simulink model "Michaels_CVModel_fast8"  (R2020a)
settings: Solver=ode23  StartTime=0.0  StopTime=30  RelTol=1e-2  EnableMultiTasking=on
model workspace (MAT data in the model file):
  Eao = 1.88
  Eesla = 0.58
  Eeslvf = 5.2
  Eesra = 0.63
  Eesrvf = 1.75
  Emaxspt = 48.75
  Epa = 0.15
  Epu = 0.04
  Esa = 0.37
  Esv = 0.013
  Evc = 0.03
  GpLV = 0
  GpRR = 11
  GpRV = 0
  GpRsa = 0
  GpV0 = 0
  GsLV = 0.007
  GsRR = 11
  GsRV = 0.022
  GsRsa = -0.05
  GsV0 = 31
  Ka = 4.4
  Lao = 0.0022
  Lav = 0.000354
  Lmt = 7.697e-05
  Lpa = 7.697e-05
  Lpv = 0.0001043
  Ltc = 8.009e-05
  P0la = 0.5
  P0lvf = 0.98
  P0pcd = 0.5
  P0ra = 0.5
  P0rvf = 0.91
  P0spt = 0.46
  PV : AO (value not decoded)
  PVao = [327.9; 100.9]
  Rao = 0.28
  Rav = 0.02
  Rla2pu = 0.5
  Rmt = 0.01
  Rpa = 0.12
  Rpa_Vals = 0.12
  Rpu = 0.006
  Rpv = 0.02
  Rra = 0.012
  Rsa = 0.74
  Rsv = 0.12
  Rtc = 0.01
  Tc = 1
  Tsys0 = 0.6
  V0la = 30
  V0lvf = 45
  V0pcd = 200
  V0ra = 25
  V0rvf = 50
  V0spt = 10
  Vdla = 15
  Vdlvf = 16
  Vdra = 15
  Vdrvf = 40
  Vdspt = 10
  Vlv0 = 100
  Vperi = 51
  Vrv0 = 105
  Vuao = 260.8
  Vupa = 91
  Vupu = 132
  Vusa = 287.4
  Vusv = 1976.1
  Vuvc = 136.17
  amin = -2
  artBrLVcontConti = []
  artBrLVcontDigi = [0 0 0 0 0 0 0 0 0 0 0 0 ... (240 elements, 1x240)]
  artBrRRConti = []
  artBrRRDigi = [0 0 0 0 0 0 0 0 0 0 1.57142857143 3.14285714286 ... (240 elements, 1x240)]
  artBrRVcontConti = []
  artBrRVcontDigi = [0 0 0 0 0 0 0 0 0 0 0 0 ... (240 elements, 1x240)]
  artBrRsaConti = []
  artBrRsaDigi = [0 0 0 0 0 0 0 0 0 0 0 0 ... (480 elements, 1x480)]
  artBrV0Conti = []
  artBrV0Digi = [0 0 0 0 0 0 0 0 0 0 0 0 ... (640 elements, 1x640)]
  atriumA = 1
  baroSampFreq = 16
  cP0la = 0.5
  cP0lvf = 0.98
  cP0ra = 0.5
  cP0rvf = 0.91
  cT = 1
  cVtotal = 5400
  clambdala = 0.13
  clambdalvf = 0.028
  clambdara = 0.13
  clambdarvf = 0.028
  deac = 0.0004
  ksys = 0.075
  lambdala = 0.065
  lambdalvf = 0.042
  lambdapcd = 0.005
  lambdara = 0.065
  lambdarvf = 0.028
  lambdaspt = 0.4
  pThor = 0
  params : object (value not decoded)
  sampleTime = 0.005
  svcPressureChange_MCS = 0
  svrMult = 1
  tStepOn = 1000000000
  t_baroOn = 1000000
  t_testBed_start = 1000000
  venk1 = 0.5
  venk2 = 0.5
symbols that are objects in the model workspace (value not decoded): PV
undefined symbols (not defined in the file): dfilt
libraries: simulink x85, fl_lib x39, nesl_utility x24, cstblocks x9, dspstat3 x9, dspobslib x5, SimscapeFluids_lib x5, sh_lib x1
(part 4 of 5)

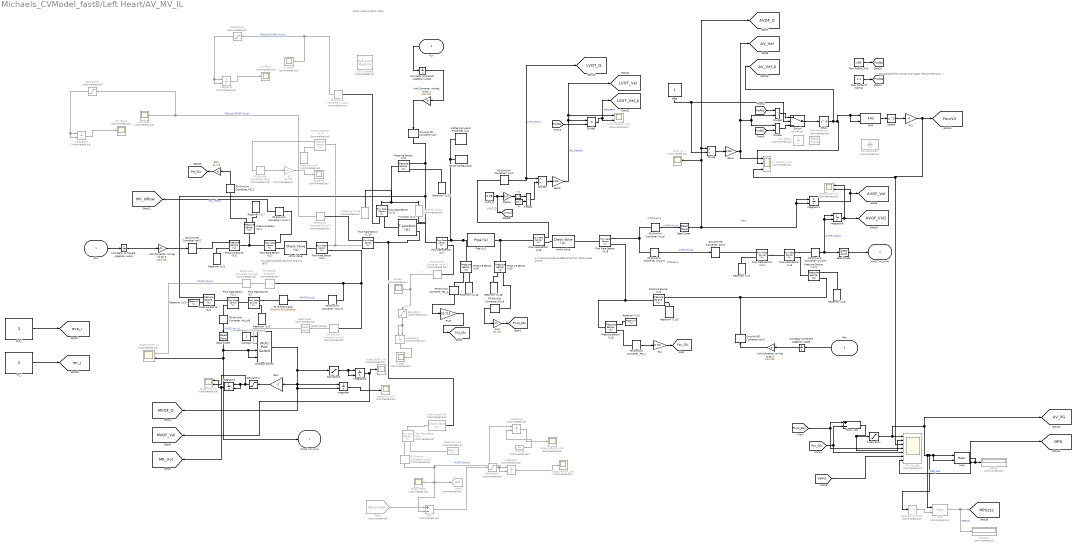
== system Michaels_CVModel_fast8/Left Heart/AV_MV_IL ==
  note: MV opening pressures from Tsakiris 1978
  note: AV cracking pressure differential from 2019 Lansac article
  note: Extrapolated from Donati 2017 paper "Beyond Bernoulli..."
  note: Filtered Q
  note: Unfiltered Q
  note: 1 = Unfiltered Q
      | 2= Filtered Q
  note: Area
  note: Aortic Valve & Mitral Valve
  PLA : Inport
  PLV : Inport  Port=2
  PAo : Inport  Port=3
  4V2 : Gain  Gain=4
  51.1 : Gain  Gain=51.715
  51.7 : Gain  Commented=on  Gain=51.715
  51.8 : Gain  Gain=51.715
  AV Velocity (m/s) : Scope  Commented=on  NumInputPorts=3
  AVOF_Q : Scope  Commented=on
  Add : Sum  Commented=on  Inputs=+-
  Aortic Valve : SimscapeFluids_lib/Isothermal Liquid/Valves & Orifices/Directional Control Valves/Check Valve (IL)  pressure_control_spec=fluids.isothermal_liquid.valves_orifices.enum.pressure_control_spec.dp  p_crack_differential=0.01 psi  p_crack_gauge=0.001 psi  press_max_differential=0.25 psi  press_max_gauge=0.002 psi  area_max=4 cm^2  area_leak=1e-13 cm^2  area=inf cm^2  Cd=0.85  Re_c=8000  pressure_recovery=simscape.enum.onoff.off  opening_dynamics=simscape.enum.onoff.on  tau=10 ms  mdot_A_specify=off  mdot_A_priority=None  mdot_A=0 kg/s  mdot_A_nominal_specify=off  mdot_A_nominal_unit=kg/s  mdot_A_nominal_value=1  mdot_B_specify=off  mdot_B_priority=None  mdot_B=0 kg/s  mdot_B_nominal_specify=off  mdot_B_nominal_unit=kg/s  mdot_B_nominal_value=1
      settings: SourceProductBaseCode=SH  InternalSimscapePortConfiguration="{\"Bottom\":[],\"Left\":[{\"id\":\"A\",\"label\":\"A\",\"type\":\"foundation.isothermal_liquid.isothermal_liquid\"}],\"Right\":[{\"id\":\"B\",\"label\":\"B\",\"type\":\"foundation.isothermal_liquid.isothermal_liquid\"}],\"Top\":[]}"
  Check Valve (MR) : SimscapeFluids_lib/Isothermal Liquid/Valves & Orifices/Directional Control Valves/Check Valve (IL)  Commented=on  pressure_control_spec=fluids.isothermal_liquid.valves_orifices.enum.pressure_control_spec.dp  p_crack_differential=0.001 psi  p_crack_gauge=0.1 MPa  press_max_differential=0.00101 psi  press_max_gauge=0.2 MPa  area_max=0.2 cm^2  area_leak=1e-13 cm^2  area=inf cm^2  Cd=0.9  Re_c=5000  pressure_recovery=simscape.enum.onoff.off  opening_dynamics=simscape.enum.onoff.off  tau=0.1 s  mdot_A_specify=off  mdot_A_priority=None  mdot_A=0 kg/s  mdot_A_nominal_specify=off  mdot_A_nominal_unit=kg/s  mdot_A_nominal_value=1  mdot_B_specify=off  mdot_B_priority=None  mdot_B=0 kg/s  mdot_B_nominal_specify=off  mdot_B_nominal_unit=kg/s  mdot_B_nominal_value=1
      settings: SourceProductBaseCode=SH  InternalSimscapePortConfiguration="{\"Bottom\":[],\"Left\":[{\"id\":\"A\",\"label\":\"A\",\"type\":\"foundation.isothermal_liquid.isothermal_liquid\"}],\"Right\":[{\"id\":\"B\",\"label\":\"B\",\"type\":\"foundation.isothermal_liquid.isothermal_liquid\"}],\"Top\":[]}"
  Compare To Zero1 : simulink/Logic and Bit Operations/Compare To Zero  Commented=on  relop=>  OutDataTypeStr=boolean
  Constant : Constant  Value=2
  Dead Zone2 : DeadZone  Commented=on  LowerValue=-0.01  UpperValue=0.01  SaturateOnIntegerOverflow=on
  Dead Zone3 : DeadZone  LowerValue=-0.001  UpperValue=0.001  ZeroCross=off  SaturateOnIntegerOverflow=on
  Dead Zone4 : DeadZone  LowerValue=-0.001  UpperValue=0.001  ZeroCross=off  SaturateOnIntegerOverflow=on
  Dead Zone5 : DeadZone  LowerValue=-0.001  UpperValue=0.001  ZeroCross=off  SaturateOnIntegerOverflow=on
  Delay : Delay  DelayLength=0  SampleTime=0.001
  Discrete Filter1 : DiscreteFilter  Commented=on  Denominator=[1]  SampleTime=0.001
  Display : Display  Commented=on
  Display1 : Display  Commented=on
  Divide : Product  Inputs=*/
  Divide1 : Product  Inputs=**
  Divide2 : Product  Inputs=*/
  Divide3 : Product  Inputs=**
  Divide4 : Product  Inputs=**
  Flow Profile Cf AS : Constant  Value=1.305  SampleTime=0.001
  Flow Profile Cf Normal : Constant  Value=1.1  SampleTime=0.001
  Flow Rate Sensor (IL){1..3,5,7..11} (9 alike) : fl_lib/Isothermal Liquid/Sensors/Flow Rate Sensor (IL)  sensor_type=foundation.enum.mass_volumetric_sensor.volumetric
      settings: SourceProductBaseCode=SS  InternalSimscapePortConfiguration="{\"Bottom\":[],\"Left\":[{\"id\":\"A\",\"label\":\"A\",\"type\":\"foundation.isothermal_liquid.isothermal_liquid\"}],\"Right\":[{\"id\":\"B\",\"label\":\"B\",\"type\":\"foundation.isothermal_liquid.isothermal_liquid\"},{\"id\":\"V\",\"label\":\"V\",\"type\":\"output\"}],\"Top\":[]}"
  Flow Rate Sensor (IL)6 : fl_lib/Isothermal Liquid/Sensors/Flow Rate Sensor (IL)  Commented=on  sensor_type=foundation.enum.mass_volumetric_sensor.volumetric
      settings: SourceProductBaseCode=SS  InternalSimscapePortConfiguration="{\"Bottom\":[],\"Left\":[{\"id\":\"A\",\"label\":\"A\",\"type\":\"foundation.isothermal_liquid.isothermal_liquid\"}],\"Right\":[{\"id\":\"B\",\"label\":\"B\",\"type\":\"foundation.isothermal_liquid.isothermal_liquid\"},{\"id\":\"V\",\"label\":\"V\",\"type\":\"output\"}],\"Top\":[]}"
  Flow Rate Source (IL) : fl_lib/Isothermal Liquid/Sources/Flow Rate Source (IL)  source_type=foundation.enum.constant_controlled.controlled  flow_type=foundation.enum.mass_volumetric_flow.volumetric  mass_flow=0 kg/s  volumetric_flow=0 m^3/s
      settings: SourceProductBaseCode=SS  InternalSimscapePortConfiguration="{\"Bottom\":[],\"Left\":[{\"id\":\"A\",\"label\":\"A\",\"type\":\"foundation.isothermal_liquid.isothermal_liquid\"},{\"id\":\"V\",\"label\":\"V\",\"type\":\"input\"}],\"Right\":[{\"id\":\"B\",\"label\":\"B\",\"type\":\"foundation.isothermal_liquid.isothermal_liquid\"}],\"Top\":[]}"
  Flow Rate Source (IL)1 : fl_lib/Isothermal Liquid/Sources/Flow Rate Source (IL)  source_type=foundation.enum.constant_controlled.controlled  flow_type=foundation.enum.mass_volumetric_flow.volumetric  mass_flow=0 kg/s  volumetric_flow=0 m^3/s
      settings: SourceProductBaseCode=SS  InternalSimscapePortConfiguration="{\"Bottom\":[],\"Left\":[{\"id\":\"A\",\"label\":\"A\",\"type\":\"foundation.isothermal_liquid.isothermal_liquid\"},{\"id\":\"V\",\"label\":\"V\",\"type\":\"input\"}],\"Right\":[{\"id\":\"B\",\"label\":\"B\",\"type\":\"foundation.isothermal_liquid.isothermal_liquid\"}],\"Top\":[]}"
  From16 : From  Commented=on  GotoTag=ev  TagVisibility=global
      settings: CloseFcn=tagdialog Close
  From2 : From  Commented=on  GotoTag=MV_Inflow  TagVisibility=global
  Gain : Gain  Gain=-1
  Gain1 : Gain  Gain=1/100
  Gain3 : Gain  Gain=1/100
  Goto3 : Goto  Commented=on  GotoTag=QMR  TagVisibility=global
  Integrator{,1..3,9} (5 alike) : Integrator  ExternalReset=either
  Integrator4 : Integrator  Commented=on  ExternalReset=either
  Integrator5 : Integrator  Commented=on  ExternalReset=either
  Integrator6 : Integrator  Commented=on  ExternalReset=rising
  Integrator7 : Integrator  Commented=on  ExternalReset=rising
  Integrator8 : Integrator  Commented=on  ExternalReset=rising
  Isothermal Liquid Properties (IL)1 : fl_lib/Isothermal Liquid/Utilities/Isothermal Liquid Properties (IL)  rho_L_atm=1107.1 kg/m^3  bulk_modulus_model=foundation.enum.bulk_modulus_model.const  beta_gain=6  beta_L_atm=2.1791e9 Pa  nu_atm=3.5 cSt  air_fraction=0  polytropic_index=1.0  rho_g_atm=1.225 kg/m^3  air_dissolution_model=simscape.enum.onoff.off  p_crit=3 MPa  p_atm=14.6959 psi  p_min=1e-13 psi
      settings: SourceProductBaseCode=SS
  LV Inflow2 : Scope  Commented=on
  LV Inflow3 : Scope  Commented=on
  LVOT Velocity (m/s) : Scope  Commented=on  NumInputPorts=2
  LVOT1 -flexible : sh_lib/Pipelines/Hydraulic Pipeline  Commented=on  cs_type=1  d_in=2.0 cm  area=1e-4 m^2  D_h=1.12e-2 m  s_factor=64  length=1.8 cm  length_ad=0.4 cm  roughness=0.1 cm  Re_lam=2000  Re_turb=5000  wall_type=2  pr_r_coef=2e-12 m/Pa  time_const=0.01 s  k_sh=1.4  initial_pressure=0.01 psi
      settings: SourceProductBaseCode=SH  InternalSimscapePortConfiguration="{\"Bottom\":[],\"Left\":[{\"id\":\"A\",\"label\":\"A\",\"type\":\"foundation.hydraulic.hydraulic\"}],\"Right\":[{\"id\":\"B\",\"label\":\"B\",\"type\":\"foundation.hydraulic.hydraulic\"}],\"Top\":[]}"
  LVOT_D : Constant  Value=2.25
  MPG : dspstat3/Mean  run=on  reset_popup=Either edge  directionMode=Each column  dimension=1  roiEnable=off  roiType=Rectangles  roiPortion=Entire ROI  roiOutput=Individual statistics for each ROI  roiFlag=off  roundingMode=Floor  overflowMode=off  outputDataTypeStr=Inherit: Same as accumulator  outputMin=[]  outputMax=[]  outputLastDataTypeStr=Inherit: Same as accumulator
  MPG1 : dspstat3/Mean  Commented=on  run=on  reset_popup=Either edge  directionMode=Each column  dimension=1  roiEnable=off  roiType=Rectangles  roiPortion=Entire ROI  roiOutput=Individual statistics for each ROI  roiFlag=off  roundingMode=Floor  overflowMode=off  outputDataTypeStr=Inherit: Same as accumulator  outputMin=[]  outputMax=[]  outputLastDataTypeStr=Inherit: Same as accumulator
  MR Inflow : Scope  Commented=on
  MR Inflow1 : Scope  Commented=on
  Mitral Valve : SimscapeFluids_lib/Isothermal Liquid/Valves & Orifices/Directional Control Valves/Check Valve (IL)  pressure_control_spec=fluids.isothermal_liquid.valves_orifices.enum.pressure_control_spec.dp  p_crack_differential=0.0001 psi  p_crack_gauge=0.001 psi  press_max_differential=0.15 psi  press_max_gauge=0.002 psi  area_max=5 cm^2  area_leak=1e-13 cm^2  area=3.1416*1.27^2 cm^2  Cd=0.85  Re_c=5000  pressure_recovery=simscape.enum.onoff.off  opening_dynamics=simscape.enum.onoff.on  tau=20 ms  mdot_A_specify=off  mdot_A_priority=None  mdot_A=0 kg/s  mdot_A_nominal_specify=off  mdot_A_nominal_unit=kg/s  mdot_A_nominal_value=1  mdot_B_specify=off  mdot_B_priority=None  mdot_B=0 kg/s  mdot_B_nominal_specify=off  mdot_B_nominal_unit=kg/s  mdot_B_nominal_value=1
      settings: SourceProductBaseCode=SH  InternalSimscapePortConfiguration="{\"Bottom\":[],\"Left\":[{\"id\":\"A\",\"label\":\"A\",\"type\":\"foundation.isothermal_liquid.isothermal_liquid\"}],\"Right\":[{\"id\":\"B\",\"label\":\"B\",\"type\":\"foundation.isothermal_liquid.isothermal_liquid\"}],\"Top\":[]}"
  Multiport Switch : MultiPortSwitch
  P saturation : Saturate  UpperLimit=inf  LowerLimit=0
  PS Transfer Function1 : fl_lib/Physical Signals/Linear Operators/PS Transfer Function  Commented=on  transfer_function_type=foundation.enum.transfer_function_type.lag  T=5 ms  T1=2 s  T2=1 s  y0=100 cm^3/s
      settings: SourceProductBaseCode=SS  InternalSimscapePortConfiguration="{\"Bottom\":[],\"Left\":[{\"id\":\"U\",\"label\":\"\",\"type\":\"input\"}],\"Right\":[{\"id\":\"Y\",\"label\":\"\",\"type\":\"output\"}],\"Top\":[]}"
  PS-Simulink Converter (mL/s){,5,7..9} (5 alike) : nesl_utility/PS-Simulink Converter  PhysicalDomain=network_engine_domain  SubClassName=ps_output  LeftPortType=input  RightPortType=output  PseudoPeriodic=off  Frequencies=[]  Unit=cm^3/s  AffineConversion=off
  "PS-Simulink Converter (mL/s) " : nesl_utility/PS-Simulink Converter  PhysicalDomain=network_engine_domain  SubClassName=ps_output  LeftPortType=input  RightPortType=output  PseudoPeriodic=off  Frequencies=[]  Unit=cm^3/s  AffineConversion=off
  PS-Simulink Converter (mL/s) 1 : nesl_utility/PS-Simulink Converter  Commented=on  PhysicalDomain=network_engine_domain  SubClassName=ps_output  LeftPortType=input  RightPortType=output  PseudoPeriodic=off  Frequencies=[]  Unit=cm^3/s  AffineConversion=off
  PS-Simulink Converter (mL/s) 2 : nesl_utility/PS-Simulink Converter  PhysicalDomain=network_engine_domain  SubClassName=ps_output  LeftPortType=input  RightPortType=output  PseudoPeriodic=off  Frequencies=[]  Unit=cm^3/s  AffineConversion=off
  PS-Simulink Converter (mL/s){1..4,6} (5 alike) : nesl_utility/PS-Simulink Converter  Commented=on  PhysicalDomain=network_engine_domain  SubClassName=ps_output  LeftPortType=input  RightPortType=output  PseudoPeriodic=off  Frequencies=[]  Unit=cm^3/s  AffineConversion=off
  PS-Simulink Converter_PSI_{1..2,4,9} (4 alike) : nesl_utility/PS-Simulink Converter  PhysicalDomain=network_engine_domain  SubClassName=ps_output  LeftPortType=input  RightPortType=output  PseudoPeriodic=off  Frequencies=[]  Unit=psi  AffineConversion=off
  PS-Simulink Converter_PSI_8 : nesl_utility/PS-Simulink Converter  Commented=on  PhysicalDomain=network_engine_domain  SubClassName=ps_output  LeftPortType=input  RightPortType=output  PseudoPeriodic=off  Frequencies=[]  Unit=psi  AffineConversion=off
  Pav : Gain  Gain=51.715
  Pi : Constant  Value=pi()  SampleTime=0.001
  Pipe (IL)1 : SimscapeFluids_lib/Isothermal Liquid/Pipes & Fittings/Pipe (IL)  dynamic_compressibility=simscape.enum.onoff.off  inertia=simscape.enum.onoff.off  num_segments=1  pipe_length=1.8 cm  cross_section_geometry=fluids.isothermal_liquid.pipes_fittings.enum.cross_section_geometry.circular  pipe_diameter=2.25 cm  pipe_inner_diameter=0.05 m  pipe_outer_diameter=0.1 m  pipe_width=0.1 m  pipe_height=0.1 m  pipe_major_axis=0.1 m  pipe_minor_axis=0.05 m  pipe_side=0.1 m  pipe_angle=30 deg  pipe_area=0.01 m^2  Dh=0.1128 m  elevation_spec=foundation.enum.constant_variable.constant  elevation_gain=0 cm  gravity_spec=foundation.enum.constant_variable.constant  g=9.81 m/s^2  pressure_loss_spec=fluids.isothermal_liquid.pipes_fittings.enum.pressure_loss_spec.haaland  mdot_nominal=[.1, 1] kg/s  p_diff_nominal=[.001, .01] MPa  mdot_threshold=1e-6 kg/s  local_pressure_loss_spec=fluids.isothermal_liquid.pipes_fittings.enum.local_loss_spec.aggregate_length  length_add=0.004 cm  loss_coefficient=0.1  roughness_spec=fluids.isothermal_liquid.pipes_fittings.enum.roughness_spec.commercial_pipe  roughness=15e-6 m  Re_friction_TLU=[400, 1000, 1500, 3000, 4000, 6000, 10000, 20000, 40000, 60000, 100000, 100000000]  friction_factor_TLU=[.264, .112, .071, .0417, .0387, .0268, .025, .0232, .0226, .022, .0214, .0214]  Re_lam=5000  Re_tur=8000  shape_factor=64  pipe_wall_spec=fluids.isothermal_liquid.pipes_fittings.enum.wall_spec.flexible  vol_expansion_spec=fluids.isothermal_liquid.pipes_fittings.enum.vol_expansion_spec.area  area_pressure_gain=0.005 m^2/MPa  diameter_pressure_gain=1e-6 m/MPa  wall_time_constant=0.12 s  p0=0.1 psi  mdot0=0 kg/s
      settings: SourceProductBaseCode=SH  InternalSimscapePortConfiguration="{\"Bottom\":[],\"Left\":[{\"id\":\"A\",\"label\":\"A\",\"type\":\"foundation.isothermal_liquid.isothermal_liquid\"}],\"Right\":[{\"id\":\"B\",\"label\":\"B\",\"type\":\"foundation.isothermal_liquid.isothermal_liquid\"}],\"Top\":[]}"
  Plv_Pav_Sat : Scope  Commented=on  NumInputPorts=7
  Plvot : Gain  Gain=51.715
  Plvot - Pav : Sum  Inputs=+-
  Pressure Sensor (IL){1,6,8..9} (4 alike) : fl_lib/Isothermal Liquid/Sensors/Pressure Sensor (IL)  pressure_measure=foundation.enum.pressure_measure.difference
      settings: SourceProductBaseCode=SS  InternalSimscapePortConfiguration="{\"Bottom\":[],\"Left\":[{\"id\":\"A\",\"label\":\"A\",\"type\":\"foundation.isothermal_liquid.isothermal_liquid\"}],\"Right\":[{\"id\":\"B\",\"label\":\"B\",\"type\":\"foundation.isothermal_liquid.isothermal_liquid\"},{\"id\":\"P\",\"label\":\"P\",\"type\":\"output\"}],\"Top\":[]}"
  Pressure Sensor (IL)5 : fl_lib/Isothermal Liquid/Sensors/Pressure Sensor (IL)  Commented=on  pressure_measure=foundation.enum.pressure_measure.difference
      settings: SourceProductBaseCode=SS  InternalSimscapePortConfiguration="{\"Bottom\":[],\"Left\":[{\"id\":\"A\",\"label\":\"A\",\"type\":\"foundation.isothermal_liquid.isothermal_liquid\"}],\"Right\":[{\"id\":\"B\",\"label\":\"B\",\"type\":\"foundation.isothermal_liquid.isothermal_liquid\"},{\"id\":\"P\",\"label\":\"P\",\"type\":\"output\"}],\"Top\":[]}"
  Pressure Source (IL){1..5} (5 alike) : fl_lib/Isothermal Liquid/Sources/Pressure Source (IL)  source_type=foundation.enum.constant_controlled.controlled  pressure_differential=0 MPa
      settings: SourceProductBaseCode=SS  InternalSimscapePortConfiguration="{\"Bottom\":[],\"Left\":[{\"id\":\"A\",\"label\":\"A\",\"type\":\"foundation.isothermal_liquid.isothermal_liquid\"},{\"id\":\"P\",\"label\":\"P\",\"type\":\"input\"}],\"Right\":[{\"id\":\"B\",\"label\":\"B\",\"type\":\"foundation.isothermal_liquid.isothermal_liquid\"}],\"Top\":[]}"
  Product : Product
  RMS : dspstat3/RMS  run=on  directionMode=Each column  dimension=1  reset_popup=Either edge
  Radius : Gain  Gain=0.5
  Rate Transition2 : RateTransition  Commented=on
  Reservoir (IL){1..7,13,15,18..19} (11 alike) : fl_lib/Isothermal Liquid/Elements/Reservoir (IL)  reservoir_type=foundation.enum.constant_controlled.constant  pressure_spec=foundation.enum.pressure_spec.atmospheric  reservoir_pressure=0.101325 MPa
      settings: SourceProductName=Foundation Library
  Reservoir (IL)11 : fl_lib/Isothermal Liquid/Elements/Reservoir (IL)  Commented=on  reservoir_type=foundation.enum.constant_controlled.controlled  pressure_spec=foundation.enum.pressure_spec.atmospheric  reservoir_pressure=0.101325 MPa
      settings: SourceProductName=Foundation Library  InternalSimscapePortConfiguration="{\"Bottom\":[],\"Left\":[{\"id\":\"A\",\"label\":\"A\",\"type\":\"foundation.isothermal_liquid.isothermal_liquid\"}],\"Right\":[{\"id\":\"P\",\"label\":\"P\",\"type\":\"input\"}],\"Top\":[]}"
  Reservoir (IL)16 : fl_lib/Isothermal Liquid/Elements/Reservoir (IL)  Commented=on  reservoir_type=foundation.enum.constant_controlled.constant  pressure_spec=foundation.enum.pressure_spec.atmospheric  reservoir_pressure=0.101325 MPa
      settings: SourceProductName=Foundation Library
  Reservoir (IL)8 : fl_lib/Isothermal Liquid/Elements/Reservoir (IL)  Commented=on  reservoir_type=foundation.enum.constant_controlled.constant  pressure_spec=foundation.enum.pressure_spec.atmospheric  reservoir_pressure=0.101325 MPa
      settings: SourceProductName=Foundation Library
  Reservoir (IL)9 : fl_lib/Isothermal Liquid/Elements/Reservoir (IL)  Commented=on  reservoir_type=foundation.enum.constant_controlled.constant  pressure_spec=foundation.enum.pressure_spec.atmospheric  reservoir_pressure=0.101325 MPa
      settings: SourceProductName=Foundation Library
  Saturation1 : Saturate  UpperLimit=inf  LowerLimit=0
  Saturation2 : Saturate  UpperLimit=inf  LowerLimit=0
  Saturation{5..7,9} (4 alike) : Saturate  Commented=on  UpperLimit=inf  LowerLimit=0
  Scope1 : Scope  Commented=on
  Scope3 : Scope  Commented=on
  Scope_AVOF_Vol : Scope  Commented=on  NumInputPorts=2
  Scope_MROF : Scope  Commented=on
  Scope_MRVOF_Vol1 : Scope  Commented=on
  Scope_MRVOF_Vol2 : Scope  Commented=on
  Scope_MR_Vol : Scope  Commented=on  NumInputPorts=2
  Scope_MVOF_Q : Scope  Commented=on  NumInputPorts=2
  Scope_MVOF_Vol : Scope  Commented=on
  Scope_MV_Vol2 : Scope  Commented=on
  Scope_P1 : Scope  Commented=on
  Simulink-PS Converter (psi) : nesl_utility/Simulink-PS Converter  PhysicalDomain=network_engine_domain  SubClassName=ps_input  LeftPortType=input  RightPortType=output  PseudoPeriodic=off  Frequencies=[]  NoiseDistribution=none  NoiseParameters=[]  Unit=psi  AffineConversion=off  FilteringAndDerivatives=filter  SimscapeFilterOrder=1  InputFilterTimeConstant=.001  UdotUserProvided=0
  Simulink-PS Converter (psi)1 : nesl_utility/Simulink-PS Converter  PhysicalDomain=network_engine_domain  SubClassName=ps_input  LeftPortType=input  RightPortType=output  PseudoPeriodic=off  Frequencies=[]  NoiseDistribution=none  NoiseParameters=[]  Unit=psi  AffineConversion=off  FilteringAndDerivatives=filter  SimscapeFilterOrder=1  InputFilterTimeConstant=.001  UdotUserProvided=0
  Simulink-PS Converter (psi)2 : nesl_utility/Simulink-PS Converter  PhysicalDomain=network_engine_domain  SubClassName=ps_input  LeftPortType=input  RightPortType=output  PseudoPeriodic=off  Frequencies=[]  NoiseDistribution=none  NoiseParameters=[]  Unit=psi  AffineConversion=off  FilteringAndDerivatives=filter  SimscapeFilterOrder=1  InputFilterTimeConstant=.001  UdotUserProvided=0
  Simulink-PS Converter (psi)5 : nesl_utility/Simulink-PS Converter  PhysicalDomain=network_engine_domain  SubClassName=ps_input  LeftPortType=input  RightPortType=output  PseudoPeriodic=off  Frequencies=[]  NoiseDistribution=none  NoiseParameters=[]  Unit=cm^3/s  AffineConversion=off  FilteringAndDerivatives=filter  SimscapeFilterOrder=1  InputFilterTimeConstant=.002  UdotUserProvided=0
  "Solver Configuration " : nesl_utility/Solver Configuration  PhysicalDomain=network_engine_domain  SubClassName=solver  LeftPortType=input  RightPortType=generic  Tones=[]  Harmonics=[]  SimulateNoise=off  Profile=off  UseLocalSampling=off  EnableSwitchedLinearOptims=on  FrequencyDomain=off  UseCCode=off  RelTol=0.001  AbsTol=1e-06  MinStep=1e-09  ToWorkspace=off  RevertToSquareIcSolve=off  NumHomotopyIterations=100  PhasorMode=off  PhasorModeNumHarmonics=1  DoDC=off  ResidualTolerance=1e-09  UseLocalSolver=on  LocalSolverChoice=NE_BACKWARD_EULER_ADVANCER  LocalSolverSampleTime=1/512  DoFixedCost=on  MaxNonlinIter=3  MaxModeIter=2  LinearAlgebra=Sparse  EquationFormulation=NE_TIME_EF  DelaysMemoryBudget=1024  AutomaticFiltering=on  FilteringTimeConstant=0.005  PartitionStorageMethod=AS_NEEDED  PartitionMemoryBudget=1024  PartitionMethod=FAST
  Square : Math  Operator=square  SaturateOnIntegerOverflow=on
  Switch : Switch  Threshold=1.5
  T-Junction (IL)1 : SimscapeFluids_lib/Isothermal Liquid/Pipes & Fittings/T-Junction (IL)  area_main=10 cm^2  area_branch=5 cm^2  junction_spec=fluids.isothermal_liquid.pipes_fittings.enum.three_way_junction_spec.custom  k_main_converge=1  k_main_diverge=1  k_branch_converge=1  k_branch_diverge=1  Re_c=5000  mdot_A_specify=off  mdot_A_priority=None  mdot_A=0 kg/s  mdot_A_nominal_specify=off  mdot_A_nominal_unit=kg/s  mdot_A_nominal_value=1  mdot_B_specify=off  mdot_B_priority=None  mdot_B=0 kg/s  mdot_B_nominal_specify=off  mdot_B_nominal_unit=kg/s  mdot_B_nominal_value=1  mdot_C_specify=off  mdot_C_priority=None  mdot_C=0 kg/s  mdot_C_nominal_specify=off  mdot_C_nominal_unit=kg/s  mdot_C_nominal_value=1
      settings: SourceProductBaseCode=SH  InternalSimscapePortConfiguration="{\"Bottom\":[{\"id\":\"C\",\"label\":\"C\",\"type\":\"foundation.isothermal_liquid.isothermal_liquid\"}],\"Left\":[{\"id\":\"A\",\"label\":\"A\",\"type\":\"foundation.isothermal_liquid.isothermal_liquid\"}],\"Right\":[{\"id\":\"B\",\"label\":\"B\",\"type\":\"foundation.isothermal_liquid.isothermal_liquid\"}],\"Top\":[]}"
  To re-filter signal : nesl_utility/Simulink-PS Converter  PhysicalDomain=network_engine_domain  SubClassName=ps_input  LeftPortType=input  RightPortType=output  PseudoPeriodic=off  Frequencies=[]  NoiseDistribution=none  NoiseParameters=[]  Unit=cm^3/s  AffineConversion=off  FilteringAndDerivatives=filter  SimscapeFilterOrder=1  InputFilterTimeConstant=.002  UdotUserProvided=0
  Unit Converter: mmHg to psi 1 : Gain  Gain=1/51.715
  Unit Converter: mmHg to psi 2 : Gain  Gain=1/51.715
  Unit Converter: mmHg to psi 3 : Gain  Gain=1/51.715
  Unit Delay to Prevent Algebraic Loop1 : UnitDelay  InitialCondition=1  SampleTime=-1  HasFrameUpgradeWarning=on
  Unit Delay to Prevent Algebraic Loop2 : UnitDelay  InitialCondition=1  SampleTime=-1  HasFrameUpgradeWarning=on
  Unit Delay to Prevent Algebraic Loop5 : UnitDelay  InitialCondition=1  SampleTime=-1  HasFrameUpgradeWarning=on
  Unit Delay1 : UnitDelay  Commented=on  SampleTime=0.005  HasFrameUpgradeWarning=on
  ^2 : Math  Operator=square  SaturateOnIntegerOverflow=on
  area : Constant  SampleTime=0.001
  ava_i : Constant  SampleTime=0.001
  mr_j : Constant  SampleTime=0.001
  MVOF [mL/min] : Outport
  AVOF [mL/min] : Outport  Port=2
  tag scope: AVOF_Q=global, AVOF_Vol2=global, AVOF_Vol=global, AV_PG=global, AV_Vel=global, AV_Vel_A=global, FourV2=global, LVOT_Q=global, LVOT_Vel=global, LVOT_Vel_A=global, Lvot_D=global, MPG=global, MPGzzz=global, MR_Vol=global, MVOF_Q=global, MVOF_Vol=global, MV_Inflow=global, PLV_SSc=global, Pav_SSc=global, Pla_SSc=global, Plvot_SSc=global, ProfAS=global, ProfNo=global, ava_i=global, mr_j=global
  wires:
  PS-Simulink Converter (mL/s) 1/1 -> Saturation7/1, Scope3/1  "]"
  Unit Converter: mmHg to psi 1/1 -> Simulink-PS Converter (psi)/1
  Unit Converter: mmHg to psi 2/1 -> Simulink-PS Converter (psi)1/1
  Pav/1 -> [Pav_SSc]
  Unit Delay to Prevent Algebraic Loop2/1 -> Unit Converter: mmHg to psi 1/1
  PS-Simulink Converter_PSI_1/1 -> Pav/1
  PLV/1 -> Unit Delay to Prevent Algebraic Loop2/1
  area/1 -> Divide/2, Switch/2
  Divide/1 -> Gain1/1
  [Plvot_SSc] -> Plv_Pav_Sat/4, Plvot - Pav/1
  [Pav_SSc] -> Plv_Pav_Sat/5, Plvot - Pav/2
  Plvot - Pav/1 -> Plv_Pav_Sat/2, P saturation/1
  Unit Converter: mmHg to psi 3/1 -> Simulink-PS Converter (psi)2/1
  PLA/1 -> Unit Delay to Prevent Algebraic Loop1/1
  Unit Delay to Prevent Algebraic Loop1/1 -> Unit Converter: mmHg to psi 3/1
  PAo/1 -> Unit Delay to Prevent Algebraic Loop5/1
  Integrator/1 -> Scope_MV_Vol2/1
  Gain/1 -> Saturation1/1
  Saturation1/1 -> Scope_MR_Vol/2, Integrator2/2, Integrator2/1
  Saturation2/1 -> Integrator3/2, Integrator3/1
  Gain1/1 -> AV Velocity (m/s)/1, Divide4/1, Divide3/2, [AV_Vel]
  "PS-Simulink Converter (mL/s) "/1 -> [LVOT_Q], Divide2/1  "LVOT_flow]"
  PS-Simulink Converter (mL/s)/1 -> Dead Zone4/1  "AVOF [mL/s]"
  Integrator1/1 -> Scope_AVOF_Vol/2, [AVOF_Vol]
  Integrator3/1 -> [MVOF_Vol], Scope_MVOF_Vol/1
  PS-Simulink Converter (mL/s)1/1 -> Dead Zone2/1  "MVOF [mL/s]"
  PS-Simulink Converter (mL/s) 2/1 -> [MV_Inflow]  "MV_Infilow"
  Integrator2/1 -> [MR_Vol], Scope_MR_Vol/1
  MPG/1 -> Plv_Pav_Sat/7, [MPG], Display/1  "MPG_end"
  PS-Simulink Converter_PSI_8/1 -> 51.7/1
  51.7/1 -> Scope_P1/1
  PS-Simulink Converter_PSI_9/1 -> 51.8/1
  PS-Simulink Converter_PSI_4/1 -> Plvot/1
  Unit Delay to Prevent Algebraic Loop5/1 -> Unit Converter: mmHg to psi 2/1
  51.8/1 -> [Plvot_SSc]
  Plvot/1 -> [PLV_SSc]
  PS-Simulink Converter (mL/s)3/1 -> MR Inflow/1, Saturation5/1  "Flow to MVMR [mL/s]"
  Saturation5/1 -> Integrator4/2, Integrator4/1
  Integrator4/1 -> MR Inflow1/1
  Integrator5/1 -> LV Inflow3/1
  Saturation6/1 -> Integrator5/1, Integrator5/2
  PS-Simulink Converter (mL/s)4/1 -> LV Inflow2/1, Saturation6/1  "Flow to MVMR [mL/s]"
  Saturation7/1 -> Integrator6/1, Integrator6/2
  Integrator6/1 -> Scope1/1
  PS-Simulink Converter (mL/s)2/1 -> Integrator8/1, Add/2, Goto3/1, Scope_MROF/1  "MVOF [mL/s]"
  Integrator7/1 -> Scope_MRVOF_Vol1/1
  From2/1 -> Add/1
  Add/1 -> Saturation9/1
  Saturation9/1 -> Integrator7/2, Integrator7/1
  From16/1 -> Integrator8/2
  Integrator8/1 -> Scope_MRVOF_Vol2/1
  ava_i/1 -> [ava_i]
  mr_j/1 -> [mr_j]
  P saturation/1 -> MPG/2, MPG/1, Compare To Zero1/1, MPG1/1, [AV_PG], Plv_Pav_Sat/1
  Compare To Zero1/1 -> MPG1/2
  MPG1/1 -> Display1/1, [MPGzzz]  "MPGzzz"
  Switch/1 -> Delay/1
  RMS/1 -> Square/1
  Square/1 -> 4V2/1
  4V2/1 -> [FourV2], AV Velocity (m/s)/3, Plv_Pav_Sat/3
  PS-Simulink Converter (mL/s)6/1 -> Scope_MVOF_Q/1  "MVOF [mL/s]"
  PS-Simulink Converter (mL/s)7/1 -> To re-filter signal/1  "MVOF [mL/s]"
  PS-Simulink Converter (mL/s)8/1 -> Dead Zone3/1  "MVOF [mL/s]"
  PS-Simulink Converter (mL/s)5/1 -> Simulink-PS Converter (psi)5/1  "AVOF [mL/s]"
  PS-Simulink Converter_PSI_2/1 -> 51.1/1
  51.1/1 -> [Pla_SSc]
  Integrator9/1 -> [AVOF_Vol2], Scope_AVOF_Vol/1
  PS-Simulink Converter (mL/s)9/1 -> Dead Zone5/1, Integrator9/2, Integrator9/1  "AVOF [mL/s]"
  Dead Zone5/1 -> AVOF [mL/min]/1
  Multiport Switch/1 -> Gain/1, Integrator/2, [MVOF_Q], Integrator/1, Saturation2/1
  Dead Zone3/1 -> Multiport Switch/4, Multiport Switch/3, MVOF [mL/min]/1, Scope_MVOF_Q/2
  Constant/1 -> Multiport Switch/1
  Dead Zone2/1 -> Multiport Switch/2
  Divide2/1 -> Gain3/1
  Gain3/1 -> [LVOT_Vel], LVOT Velocity (m/s)/1, Divide1/1  "PG_Velocity"
  Flow Profile Cf AS/1 -> [ProfAS]
  Flow Profile Cf Normal/1 -> [ProfNo]
  [ProfNo] -> Divide1/2
  [ProfNo] -> Divide3/1
  Divide3/1 -> Switch/1
  [ProfAS] -> Divide4/2
  Divide4/1 -> Switch/3
  Divide1/1 -> [LVOT_Vel_A], LVOT Velocity (m/s)/2  "AdjustedV"
  [Vel4V2] -> Plv_Pav_Sat/6
  Delay/1 -> AV Velocity (m/s)/2, RMS/2, RMS/1, [AV_Vel_A]
  Dead Zone4/1 -> Integrator1/1, Integrator1/2, [AVOF_Q], Divide/1, AVOF_Q/1
  LVOT_D/1 -> [Lvot_D], Radius/1  "LVOT_D"
  Radius/1 -> ^2/1
  ^2/1 -> Product/1
  Pi/1 -> Product/2
  Product/1 -> Divide2/2
  connections:
  Pressure Source (IL)5/LConn2 -- Pressure Source (IL)3/LConn2 -- Simulink-PS Converter (psi)1/RConn1
  PS-Simulink Converter_PSI_1/LConn1 -- Pressure Sensor (IL)8/RConn2
  PS-Simulink Converter (mL/s)7/LConn1 -- PS Transfer Function1/LConn1 -- Flow Rate Sensor (IL)5/RConn2 -- PS-Simulink Converter (mL/s)1/LConn1
  PS-Simulink Converter (mL/s) 2/LConn1 -- Flow Rate Sensor (IL)2/RConn2
  Flow Rate Sensor (IL)6/LConn1 -- Check Valve (MR)/RConn1
  Simulink-PS Converter (psi)2/RConn1 -- Pressure Source (IL)2/LConn2
  Reservoir (IL)1/LConn1 -- Pressure Source (IL)2/LConn1
  Pressure Source (IL)2/RConn1 -- Flow Rate Sensor (IL)2/LConn1 -- Pressure Sensor (IL)1/LConn1
  Flow Rate Sensor (IL)2/RConn1 -- Mitral Valve/LConn1
  Pressure Sensor (IL)5/RConn2 -- PS-Simulink Converter_PSI_8/LConn1
  Reservoir (IL)8/LConn1 -- Pressure Sensor (IL)5/RConn1
  T-Junction (IL)1/RConn2 -- Flow Rate Sensor (IL)10/LConn1 -- Check Valve (MR)/LConn1
  Flow Rate Sensor (IL)6/RConn2 -- PS-Simulink Converter (mL/s)2/LConn1
  Reservoir (IL)9/LConn1 -- Flow Rate Sensor (IL)6/RConn1
  Simulink-PS Converter (psi)/RConn1 -- Pressure Source (IL)1/LConn2 -- Reservoir (IL)11/RConn1 -- Pressure Source (IL)4/LConn2
  Pressure Source (IL)4/RConn1 -- Flow Rate Sensor (IL)11/LConn1 -- Reservoir (IL)16/LConn1 -- Reservoir (IL)11/LConn1
  T-Junction (IL)1/RConn1 -- Flow Rate Sensor (IL)7/LConn1
  Flow Rate Sensor (IL)7/RConn2 -- PS-Simulink Converter (mL/s) 1/LConn1
  Pressure Sensor (IL)6/LConn1 -- Isothermal Liquid Properties (IL)1/RConn1 -- "Solver Configuration "/RConn1 -- Flow Rate Sensor (IL)7/RConn1 -- Pipe (IL)1/LConn1
  Reservoir (IL)15/LConn1 -- Pressure Sensor (IL)6/RConn1
  Pipe (IL)1/RConn1 -- Flow Rate Sensor (IL)8/LConn1 -- Pressure Sensor (IL)9/LConn1
  Flow Rate Sensor (IL)8/RConn2 -- "PS-Simulink Converter (mL/s) "/LConn1
  Flow Rate Sensor (IL)9/RConn2 -- PS-Simulink Converter (mL/s)/LConn1 -- PS-Simulink Converter (mL/s)5/LConn1
  Pressure Source (IL)5/LConn1 -- Reservoir (IL)13/LConn1
  Pressure Source (IL)5/RConn1 -- Pressure Sensor (IL)8/LConn1 -- Flow Rate Sensor (IL)9/RConn1
  Flow Rate Sensor (IL)8/RConn1 -- Aortic Valve/LConn1
  Pressure Sensor (IL)8/RConn1 -- Reservoir (IL)5/LConn1
  Mitral Valve/RConn1 -- Flow Rate Sensor (IL)5/LConn1
  Flow Rate Sensor (IL)9/LConn1 -- Aortic Valve/RConn1
  Pressure Sensor (IL)6/RConn2 -- PS-Simulink Converter_PSI_4/LConn1
  Pressure Sensor (IL)9/RConn2 -- PS-Simulink Converter_PSI_9/LConn1
  Pressure Sensor (IL)9/RConn1 -- Reservoir (IL)18/LConn1
  Reservoir (IL)19/LConn1 -- Pressure Source (IL)4/LConn1
  Pressure Sensor (IL)5/LConn1 -- Flow Rate Sensor (IL)10/RConn1 -- Flow Rate Sensor (IL)5/RConn1
  Flow Rate Sensor (IL)10/RConn2 -- PS-Simulink Converter (mL/s)3/LConn1
  Flow Rate Sensor (IL)11/RConn1 -- T-Junction (IL)1/LConn1
  Flow Rate Sensor (IL)11/RConn2 -- PS-Simulink Converter (mL/s)4/LConn1
  Flow Rate Sensor (IL)1/RConn1 -- Pressure Source (IL)1/RConn1
  PS Transfer Function1/RConn1 -- PS-Simulink Converter (mL/s)6/LConn1
  Flow Rate Sensor (IL)1/RConn2 -- PS-Simulink Converter (mL/s)8/LConn1
  Reservoir (IL)3/LConn1 -- Pressure Source (IL)1/LConn1
  Flow Rate Source (IL)/LConn2 -- To re-filter signal/RConn1
  Flow Rate Source (IL)/RConn1 -- Flow Rate Sensor (IL)1/LConn1
  Reservoir (IL)2/LConn1 -- Flow Rate Source (IL)/LConn1
  Pressure Source (IL)3/LConn1 -- Reservoir (IL)6/LConn1
  Flow Rate Sensor (IL)3/RConn1 -- Pressure Source (IL)3/RConn1
  Flow Rate Sensor (IL)3/RConn2 -- PS-Simulink Converter (mL/s)9/LConn1
  Flow Rate Source (IL)1/RConn1 -- Flow Rate Sensor (IL)3/LConn1
  Reservoir (IL)4/LConn1 -- Flow Rate Source (IL)1/LConn1
  Flow Rate Source (IL)1/LConn2 -- Simulink-PS Converter (psi)5/RConn1
  Pressure Sensor (IL)1/RConn1 -- Reservoir (IL)7/LConn1
  Pressure Sensor (IL)1/RConn2 -- PS-Simulink Converter_PSI_2/LConn1

== system Michaels_CVModel_fast8/Stroke Work Calcs/SW Logging ==
  Mux1 : Mux  Inputs=13
  RSW_Frac : Product  Inputs=*/
  SW Logging All : Scope  Commented=on
  tswVol_j : Sum
  tag scope: J_vol_SW=global, RSW_frac=global
  wires:
  [FSW_Vol] -> Mux1/4  "FSW_Vol"
  [Pw_tsw] -> Mux1/3  "Pw_TSW"
  [TSW] -> Mux1/1  "TSW"
  [J_fsw] -> Mux1/5  "J_FSW_vol"
  [RSW_Vol] -> Mux1/8  "RSW_Vol"
  [J_tsw] -> Mux1/2  "J_TSW"
  [FSW_Q] -> Mux1/7  "FSW_Q"
  [J_rsw] -> Mux1/9  "J_RSW_vol"
  [Pw_fsw] -> Mux1/6  "Pw_FSW_vol"
  [RSW_Q] -> Mux1/11  "RSW_Q"
  [Pw_rsw] -> Mux1/10  "Pw_RSW_vol"
  [TSW_Q] -> Mux1/12  "TSWQ_av+mr"
  [TSW_Vol] -> Mux1/13  "TSWvol_av+mr"
  Mux1/1 -> SW Logging All/1
  [J_rsw] -> RSW_Frac/1
  [J_rsw] -> tswVol_j/1
  [J_fsw] -> tswVol_j/2
  tswVol_j/1 -> RSW_Frac/2, [J_vol_SW]  "TSWvol_J"
  RSW_Frac/1 -> [RSW_frac]  "RSW_frac"

== system Michaels_CVModel_fast8/Stroke Work Calcs/Stroke Work Calc AVOF ==
  Pressure : Inport
  Volume : Inport  Port=2
  Heart Rate : Inport  Port=3
  MRreg : Inport  Port=4
  2a1 : simulink/Math Operations/MinMax Running Resettable  Description=2a  Function=max  vinit=0
  Data Type Conversion : DataTypeConversion
  Demux : Demux  Outputs=3
  Derivative : Derivative
  Divide : Product  Inputs=*/
  Frequency : Gain  Gain=1/60
  Gain1 : Gain  Gain=0.5
  Memory1 : Memory
  Memory2 : Memory
  Memory3 : Memory  InheritSampleTime=on
  Memory4 : Memory
  Mux : Mux  Inputs=3
  Period : Math  Operator=reciprocal  SignedPower=on  SaturateOnIntegerOverflow=on
  Product1 : Product  RndMeth=Zero
  Product4 : Product  RndMeth=Zero
  Pulse Generator3 : DiscretePulseGenerator  PulseType=Time based  Period=20  PhaseDelay=98.7
  SW AVOF Vol : Scope  Commented=on  NumInputPorts=3
  Saturation : Saturate  UpperLimit=1  LowerLimit=0
  Scope : Scope  Commented=on  NumInputPorts=2
  Subtract1 : Sum  Inputs=+-
  Subtract2 : Sum  Inputs=+-+
  Switch : Switch  Threshold=0.5
  Triggered Subsystem : Subsystem  TreatAsAtomicUnit=on
  energy : Gain  Gain=133.3/1e6
  gain1 : Gain
  gain2 : Gain
  one1 : Constant
  zero_energy : Constant  Value=0
  Energy (Joules) : Outport  VectorParamsAs1DForOutWhenUnconnected=off
  Power (Watts) : Outport  Port=2  VectorParamsAs1DForOutWhenUnconnected=off
  Stroke Work (mmHg*mL) : Outport  Port=3  VectorParamsAs1DForOutWhenUnconnected=off
  wires:
  Triggered Subsystem/2(Out2) -> Mux/3  "End"
  Pressure/1 -> Product4/1, Memory1/1
  Volume/1 -> Memory4/1, Product1/2
  Memory4/1 -> Product4/2
  Product1/1 -> Subtract2/1  "PxV"
  Product4/1 -> Subtract2/2  "VxP"
  Memory1/1 -> Product1/1
  Subtract2/1 -> SW AVOF Vol/2, Memory2/1, Gain1/1  "SW"
  Gain1/1 -> SW AVOF Vol/1, energy/1, SW AVOF Vol/3, Triggered Subsystem/2(In2)
  energy/1 -> Triggered Subsystem/1(In1)
  Switch/1 -> Subtract2/3  "Filtered"
  zero_energy/1 -> Switch/3
  Memory2/1 -> Switch/1
  Triggered Subsystem/1(Out1) -> gain2/1, Divide/1
  Divide/1 -> gain1/1
  Memory3/1 -> Triggered Subsystem/Trigger, Data Type Conversion/1
  Derivative/1 -> Saturation/1
  one1/1 -> Subtract1/1
  Saturation/1 -> Subtract1/2
  Subtract1/1 -> Switch/2
  Data Type Conversion/1 -> Derivative/1
  Heart Rate/1 -> Frequency/1
  Frequency/1 -> Period/1
  Period/1 -> Divide/2
  MRreg/1 -> Memory3/1  "MRreg"
  Pulse Generator3/1 -> 2a1/2
  gain2/1 -> Mux/1  "End"
  gain1/1 -> Mux/2
  Mux/1 -> Scope/2, 2a1/1
  2a1/1 -> Scope/1, Demux/1
  Demux/1 -> Energy (Joules)/1
  Demux/2 -> Power (Watts)/1
  Demux/3 -> Stroke Work (mmHg*mL)/1

== system Michaels_CVModel_fast8/Stroke Work Calcs/Stroke Work MR_Vol ==
  Pressure : Inport
  Volume : Inport  Port=2
  Heart Rate : Inport  Port=3
  MRreg : Inport  Port=4
  2a1 : simulink/Math Operations/MinMax Running Resettable  Description=2a  Function=max  vinit=0
  Data Type Conversion : DataTypeConversion
  Demux : Demux  Outputs=3
  Derivative : Derivative
  Divide : Product  Inputs=*/
  Frequency : Gain  Gain=1/60
  Gain1 : Gain  Gain=0.5
  Memory1 : Memory
  Memory2 : Memory
  Memory3 : Memory  InheritSampleTime=on
  Memory4 : Memory
  Mux : Mux  Inputs=3
  Period : Math  Operator=reciprocal  SignedPower=on  SaturateOnIntegerOverflow=on
  Product1 : Product  RndMeth=Zero
  Product4 : Product  RndMeth=Zero
  Pulse Generator3 : DiscretePulseGenerator  PulseType=Time based  Period=20  PhaseDelay=98.7
  Saturation : Saturate  UpperLimit=1  LowerLimit=0
  Scope : Scope  Commented=on  NumInputPorts=2
  Subtract1 : Sum  Inputs=+-
  Subtract2 : Sum  Inputs=+-+
  Switch : Switch  Threshold=0.5
  Triggered Subsystem : Subsystem  TreatAsAtomicUnit=on
  energy : Gain  Gain=133.3/1e6
  gain1 : Gain
  gain2 : Gain
  gain3 : Gain
  one1 : Constant
  zero_energy : Constant  Value=0
  Energy (Joules) : Outport  VectorParamsAs1DForOutWhenUnconnected=off
  Power (Watts) : Outport  Port=2  VectorParamsAs1DForOutWhenUnconnected=off
  Stroke Work (mmHg*mL) : Outport  Port=3  VectorParamsAs1DForOutWhenUnconnected=off
  wires:
  Triggered Subsystem/2(Out2) -> gain3/1  "End"
  Pressure/1 -> Product4/1, Memory1/1
  Volume/1 -> Memory4/1, Product1/2
  Memory4/1 -> Product4/2
  Product1/1 -> Subtract2/1  "PxV"
  Product4/1 -> Subtract2/2  "VxP"
  Memory1/1 -> Product1/1
  Subtract2/1 -> Gain1/1, Memory2/1  "SW"
  Gain1/1 -> energy/1, Triggered Subsystem/2(In2)
  energy/1 -> Triggered Subsystem/1(In1)
  Switch/1 -> Subtract2/3  "Filtered"
  zero_energy/1 -> Switch/3
  Memory2/1 -> Switch/1
  Triggered Subsystem/1(Out1) -> gain2/1, Divide/1
  Divide/1 -> gain1/1
  Memory3/1 -> Data Type Conversion/1
  Derivative/1 -> Saturation/1
  one1/1 -> Subtract1/1
  Saturation/1 -> Subtract1/2
  Subtract1/1 -> Switch/2
  Data Type Conversion/1 -> Derivative/1
  Heart Rate/1 -> Frequency/1
  Frequency/1 -> Period/1
  Period/1 -> Divide/2
  MRreg/1 -> Triggered Subsystem/Trigger, Memory3/1  "MRreg"
  Demux/1 -> Energy (Joules)/1
  Demux/3 -> Stroke Work (mmHg*mL)/1
  gain3/1 -> Mux/3  "End"
  Pulse Generator3/1 -> 2a1/2
  Mux/1 -> 2a1/1, Scope/2
  gain1/1 -> Mux/2
  gain2/1 -> Mux/1
  2a1/1 -> Demux/1, Scope/1
  Demux/2 -> Power (Watts)/1

== system Michaels_CVModel_fast8/Stroke Work Calcs/Stroke Work Q_AV ==
  Plv : Inport
  Pao : Inport  Port=2
  Qav : Inport  Port=3
  2a1 : simulink/Math Operations/MinMax Running Resettable  Description=2a  Function=max  vinit=0
  If4 : If  IfExpression=u1 == 1  ShowElse=off
  Pulse Generator3 : DiscretePulseGenerator  PulseType=Time based  Period=20  PhaseDelay=98.7
  Relational Operator8 : RelationalOperator  Operator=>  OutDataTypeStr=boolean  RndMeth=Simplest
  Scope : Scope  Commented=on  NumInputPorts=2
  Stroke Work Action : Subsystem  TreatAsAtomicUnit=on
  Triggered Subsystem1 : Subsystem  Commented=on  TreatAsAtomicUnit=on
  FSW Q_AV : Outport
  tag scope: fswqav=global
  wires:
  2a1/1 -> Scope/1, FSW Q_AV/1, [fswqav]  "End"
  Qav/1 -> Stroke Work Action/3(Inport2)
  Plv/1 -> Relational Operator8/1, Stroke Work Action/1(In1)
  Pao/1 -> Relational Operator8/2
  If4/1 -> Stroke Work Action/Action
  Relational Operator8/1 -> Stroke Work Action/2(In2), If4/1
  Stroke Work Action/1(Outport) -> Scope/2, 2a1/1
  Pulse Generator3/1 -> 2a1/2

== system Michaels_CVModel_fast8/Stroke Work Calcs/Stroke Work Q_MR ==
  note: Need to subtract lvedp*MRvol to get area within loop
  Plv : Inport
  QMR : Inport  Port=2
  MRreg : Inport  Port=3
  meanEDP : Inport  Port=4
  MR_Vol : Inport  Port=5
  2a1 : simulink/Math Operations/MinMax Running Resettable  Description=2a  Function=max  vinit=0
  Add1 : Sum  Inputs=+-
  If4 : If  IfExpression=u1 == 1  ShowElse=off
  MR Stroke Work Action : Subsystem  TreatAsAtomicUnit=on
  Memory4 : Memory
  Product1 : Product
  Pulse Generator3 : DiscretePulseGenerator  PulseType=Time based  Period=20  PhaseDelay=98.7
  RSW_Q : Scope  Commented=on  NumInputPorts=4
  Triggered Subsystem1 : Subsystem  Commented=on  TreatAsAtomicUnit=on
  RSW Q : Outport
  tag scope: Rswqmr=global
  wires:
  2a1/1 -> RSW Q/1, [Rswqmr], RSW_Q/1  "End"
  If4/1 -> MR Stroke Work Action/Action
  Plv/1 -> MR Stroke Work Action/1(PLV)
  MRreg/1 -> MR Stroke Work Action/3(MRreg), Memory4/1  "MRreg"
  MR Stroke Work Action/1(Outport) -> RSW_Q/3, Add1/1
  Memory4/1 -> If4/1
  Product1/1 -> RSW_Q/4, Add1/2  "lvedp*MRvol"
  meanEDP/1 -> Product1/1
  MR_Vol/1 -> Product1/2  "MRreg"
  QMR/1 -> MR Stroke Work Action/2(QMR)
  Add1/1 -> 2a1/1, RSW_Q/2
  Pulse Generator3/1 -> 2a1/2

== system Michaels_CVModel_fast8/Stroke Work Calcs/Total Stroke Work LV ==
  Pressure : Inport
  Volume : Inport  Port=2
  Heart Rate : Inport  Port=3
  Lreg : Inport  Port=4
  Data Type Conversion : DataTypeConversion
  Derivative : Derivative
  Divide : Product  Inputs=*/
  Frequency : Gain  Gain=1/60
  Memory1 : Memory
  Memory2 : Memory
  Memory3 : Memory  InheritSampleTime=on
  Memory4 : Memory
  Period : Math  Operator=reciprocal  SignedPower=on  SaturateOnIntegerOverflow=on
  Product1 : Product  RndMeth=Zero
  Product4 : Product  RndMeth=Zero
  Saturation : Saturate  UpperLimit=1  LowerLimit=0
  Subtract1 : Sum  Inputs=+-
  Subtract2 : Sum  Inputs=+-+
  Switch : Switch  Threshold=0.5
  Triggered Subsystem : Subsystem  TreatAsAtomicUnit=on
  energy1 : Gain  Gain=133.3/1e6
  gain1 : Gain  Gain=-1
  gain2 : Gain  Gain=-1
  gain3 : Gain  Gain=-1
  one1 : Constant
  true_area : Gain  Gain=0.5
  zero_energy : Constant  Value=0
  Energy (Joules) : Outport  VectorParamsAs1DForOutWhenUnconnected=off
  Power (Watts) : Outport  Port=2  VectorParamsAs1DForOutWhenUnconnected=off
  Stroke Work (mmHg*mL) : Outport  Port=3  VectorParamsAs1DForOutWhenUnconnected=off
  tag scope: SW_LV=global, SWlvJ=global, SWlvP=global
  wires:
  gain3/1 -> Stroke Work (mmHg*mL)/1, [SW_LV]
  Triggered Subsystem/2(Out2) -> gain3/1
  Lreg/1 -> Memory3/1, Triggered Subsystem/Trigger  "LReg"
  Period/1 -> Divide/2
  Frequency/1 -> Period/1
  Heart Rate/1 -> Frequency/1
  Data Type Conversion/1 -> Derivative/1
  Subtract1/1 -> Switch/2
  Saturation/1 -> Subtract1/2
  one1/1 -> Subtract1/1
  Derivative/1 -> Saturation/1
  Memory3/1 -> Data Type Conversion/1
  gain1/1 -> Power (Watts)/1, [SWlvP]
  gain2/1 -> Energy (Joules)/1, [SWlvJ]  "End"
  Divide/1 -> gain1/1
  Triggered Subsystem/1(Out1) -> gain2/1, Divide/1
  Memory2/1 -> Switch/1
  zero_energy/1 -> Switch/3
  Switch/1 -> Subtract2/3  "Filtered"
  energy1/1 -> Triggered Subsystem/1(In1)
  true_area/1 -> energy1/1, Triggered Subsystem/2(In2)
  Subtract2/1 -> true_area/1, Memory2/1  "SW"
  Memory1/1 -> Product1/1
  Product4/1 -> Subtract2/2  "VxP"
  Product1/1 -> Subtract2/1  "PxV"
  Memory4/1 -> Product4/2
  Volume/1 -> Product1/2, Memory4/1
  Pressure/1 -> Memory1/1, Product4/1

== system Michaels_CVModel_fast8/Systemic/PV-aorta ==
  V : Inport
  Add1 : Sum  Inputs=-+
  Constant : Constant  Value=Vuao
  Gain : Gain  Gain=1.04
  Manual Switch : ManualSwitch
  PV aorta : Lookup_n-D  Commented=on  NumberOfTableDimensions=1  BreakpointsForDimension1=PV.AO.v  IndexSearchMethod=Linear search  BeginIndexSearchUsingPreviousIndexResult=on  Table=PV.AO.p  RndMeth=Simplest  InputSameDT=on
  P : Outport
  wires:
  V/1 -> PV aorta/1, Add1/2
  Gain/1 -> Manual Switch/1
  Manual Switch/1 -> P/1
  PV aorta/1 -> Manual Switch/2
  Constant/1 -> Add1/1
  Add1/1 -> Gain/1

== system Michaels_CVModel_fast8/Thoracic Pressure And Breathing/Breathing sinusoidal ==
  Add : Sum
  Add1 : Sum
  Constant2 : Constant  Value=10
  Constant4 : Constant  Value=0.45
  Constant5 : Constant  Value=1.21
  Constant6 : Constant  Value=3
  Divide : Product  Inputs=*/
  Divide1 : Product  Inputs=**/
  Gain : Gain  Gain=2*pi()
  Sin(2pi*t/Tresp) : Sin  TimeSource=Use external signal  SampleTime=0
  Out1 : Outport
  tag scope: Aresp=global, Bresp=global, Cresp=global, Tresp=global
  wires:
  [tt] -> Gain/1
  Gain/1 -> Divide/1
  Constant2/1 -> [Tresp]
  [Tresp] -> Divide/2
  Divide/1 -> Sin(2pi*t/Tresp)/1
  Sin(2pi*t/Tresp)/1 -> Add/1, Divide1/2  "sin(2pi*t/Tresp)"
  Constant4/1 -> [Aresp]
  Constant5/1 -> [Bresp]
  Constant6/1 -> [Cresp]
  [Bresp] -> Add/2
  Add/1 -> Divide1/3
  [Aresp] -> Divide1/1
  Divide1/1 -> Add1/1
  [Cresp] -> Add1/2
  Add1/1 -> Out1/1

== system Michaels_CVModel_fast8/Variables to Workspace/Flow ==
  Demux : Demux  Outputs=14
  L/min1 : Gain  Gain=0.06
  Mux1 : Mux  Inputs=14
  To Workspace1 : ToWorkspace  VariableName=Q_TC_V  SampleTime=0.005
  To Workspace2 : ToWorkspace  VariableName=Q_PA_V  SampleTime=0.005
  To Workspace26 : ToWorkspace  VariableName=Q_AOV  SampleTime=0.005
  To Workspace28 : ToWorkspace  VariableName=Q_AO  SampleTime=0.005
  To Workspace3 : ToWorkspace  VariableName=Q_RV  SampleTime=0.005
  To Workspace31 : ToWorkspace  VariableName=Q_SV  SampleTime=0.005
  To Workspace32 : ToWorkspace  VariableName=Q_PV  SampleTime=0.005
  To Workspace33 : ToWorkspace  VariableName=Q_PA  SampleTime=0.005
  To Workspace34 : ToWorkspace  VariableName=Q_PU  SampleTime=0.005
  To Workspace36 : ToWorkspace  VariableName=Q_MT_V  SampleTime=0.005
  To Workspace45 : ToWorkspace  VariableName=Q_RA  SampleTime=0.005
  To Workspace46 : ToWorkspace  VariableName=Q_SA  SampleTime=0.005
  To Workspace52 : ToWorkspace  VariableName=Q_LV  SampleTime=0.005
  To Workspace53 : ToWorkspace  VariableName=Q_WK  SampleTime=0.005
  wires:
  [Qav] -> Mux1/1  "Q_AoV"
  [Qao] -> Mux1/2  "Q_AO"
  [Qsv] -> Mux1/3  "Q_SV"
  [Qpv] -> Mux1/4  "Q_PV"
  [Qpa] -> Mux1/5  "Q_PA"
  [Qpu] -> Mux1/6  "Q_PU"
  [Qmt] -> Mux1/7  "Q_MT_V"
  Mux1/1 -> L/min1/1
  L/min1/1 -> Demux/1
  Demux/2 -> To Workspace28/1
  Demux/3 -> To Workspace31/1
  Demux/4 -> To Workspace32/1
  Demux/5 -> To Workspace33/1
  Demux/6 -> To Workspace34/1
  Demux/1 -> To Workspace26/1
  Demux/7 -> To Workspace36/1
  [Qra] -> Mux1/8
  [Qsa] -> Mux1/9
  [dVlvdt] -> Mux1/10
  [Qwk] -> Mux1/11
  Demux/8 -> To Workspace45/1
  Demux/9 -> To Workspace46/1
  Demux/10 -> To Workspace52/1
  Demux/11 -> To Workspace53/1
  [Qtc] -> Mux1/12
  [Qpv] -> Mux1/13
  Demux/12 -> To Workspace1/1
  Demux/13 -> To Workspace2/1
  [dVrvdt] -> Mux1/14
  Demux/14 -> To Workspace3/1
